simulink model "hexa_tilted_SOF_ANSFT"  (R2023a)
settings: Solver=ode4  StartTime=0.0  StopTime=72  FixedStep=0.01  RelTol=1e-3
model workspace (MAT data in the model file):
  hover_2m = [0  0  0  0  0  0; 0  0  0  0  0  0; 2  2  2  2  2  2; 0  0  0  0  0  0; 0  0  0  0  0  0; 0  0  0  0  0  0]
  square = [0  0  0  0  0  0; 0  0  0  0  0  0; 2.5  2.5  2.5  2.5  2.5  0; 0  0  0  0  0  0; 0  0  0  0  0  0; 0  0  0  0  0  0]
  tf = Simulink.Parameter
  tf.Value = 60
  tf.DataType = 'auto'
  tf.Complexity = 'real'
  tf.Dimensions = [1 1]
  tray0 = [0  0  0  0  0  0; 0  0  0  0  0  0; 0  5  5  5  5  0; 0  0  0  0  0  0; 0  0  0  0  0  0; 0  0  0  0  0  0]
  tray1 = [0  0  0  0  0  0; 0  0  0  0  0  0; 0  2  1  -1  1  2; 0  0  0  0  0  0; 0  0  0  0  0  0; 0  0  0  0  0  0]
  tray2 = [0  2  2  -2  -2  0; 0  0  -2  -2  2  0; 0  2  2  2  2  0; 0  0  0  0  0  0; 0  0  0  0  0  0; 0  0  0  0  0  0]
  tray3 = [0  2  2  -2  -2  0; 0  0  -2  -2  2  0; 0  2.5  2.5  2.5  2.5  0; 0  0  0  0  0  0; 0  0  0  0  0  0; 0  0  0.785  1.042  0.785  0]
  tray5 = [0  0  0  0  0  0; 0  0  0  0  0  0; 0  5  2.5  5  2.5  0; 0  0.15  0.15  0  0  0; 0  0  0.15  0.15  0  0; 0  0  0  0  0  0]
  tray_yaw = [0  0  0  0  0  0; 0  0  0  0  0  0; 0  5  2.5  5  2.5  0; 0  0  0  0  0  0; 0  0  0  0  0  0; 0  0  0.785  1.57  1.57  0.785]
  tray_yaw2 = [0  2  2  2  2  0; 0  0  0  0  0  0; 0  0  0  0  0  0; 0  0  0  0  0  0; 0  0  0  0  0  0; 0.785  0.785  1.042  1.042  0.785  0.785]
  tray_yaw3 = [0  2  2  2  2  0; 0  0  0  0  0  0; 0  0  0  0  0  0; 0  0  0  0  0  0; 0  0  0  0  0  0; 1.57079632679  1.57079632679  1.57079632679  1.57079632679  1.57079632679  1.57079632679]
  z_test = [0  0  0  0  0  0; 0  0  0  0  0  0; 0  1  2  1  1.5  2.25; 0  0  0  0  0  0; 0  0  0  0  0  0; 0  0  0  0  0  0]
undefined symbols (not defined in the file or in its folder): F, Light, MIL
libraries: dspsrcs4 x12, simulink x6, robotcorelib x2, aerolibatmos2 x2, sensorgpslib x1, mspsensorlib x1, sharedtransform x1, aerolibwind2 x1, SignalEditorBlockLib x1
settings Model: Creator=adan  LastModifiedBy=adan
settings OptimizationCC: DefaultParameterBehavior=Inlined  EnhancedBackFolding=on  PassReuseOutputArgsAs=Individual arguments  ZeroExternalMemoryAtStartup=off  ZeroInternalMemoryAtStartup=off  OptimizeBlockOrder=speed  DifferentSizesBufferReuse=on  OptimizationCustomize=off  EfficientTunableParamExpr=on
settings DebuggingCC: ParameterTunabilityLossMsg=error
settings SFSimCC: MATLABDynamicMemAlloc=off
settings RTWCC: Description=Embedded Coder  SystemTargetFile=ert.tlc  TemplateMakefile=ert_default_tmf
settings CodeAppCC: ForceParamTrailComments=on  IgnoreCustomStorageClasses=off  OperatorAnnotations=on  SimulinkDataObjDesc=on  SFDataObjDesc=on  InsertBlockDesc=on
settings ERTTargetCC: TargetLangStandard=C99 (ISO)  GenerateSampleERTMain=on  InlinedParameterPlacement=NonHierarchical  ERTCustomFileTemplate=example_file_process.tlc

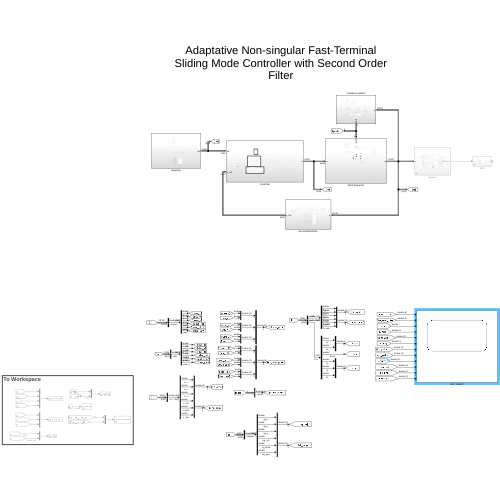
[thumbnail: Simulink's stored preview of the top-level diagram]
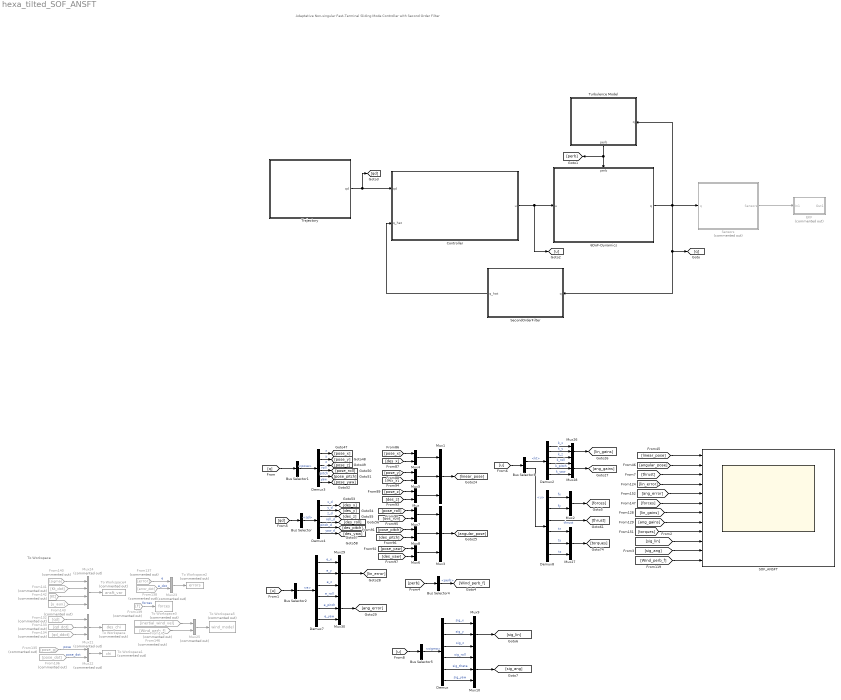
== system hexa_tilted_SOF_ANSFT ==
  note: To Workspace
  note: Adaptative Non-singular Fast-Terminal Sliding Mode Controller with Second Order Filter
  6DoF-Dynamics : Subsystem
      settings: PortSchema="{\"entries\":[{\"content\":{\"sides\":[{\"content\":{\"connectorIds\":[\"In1\"]},\"type\":\"ConnectorPlacement.EquallySpacedRectSide\",\"uuid\":\"d79ec49c-5563-41e0-ac59-6e897bc19fda\"},{\"content\":{\"connectorIds\":[\"Out1\"],\"side\":\"RIGHT\"},\"type\":\"ConnectorPlacement.EquallySpacedRectSide\",\"uuid\":\"1255043e-c90e-4bae-9fb4-4fa06f36f53e\"},{\"content\":{\"connectorIds\":[\"In2\"],\"side\":\"TOP\"},\"type\":\"ConnectorPlacement.EquallySpacedRectSide\",\"uuid\":\"823ada36-3f22-4ee3-87a1-180276f622bc\"}]},\"type\":\"ConnectorPlacement.EquallySpacedConnector\",\"uuid\":\"7403b609-b333-4977-a854-ed7a71f74338\"}],\"packageUris\":[\"http://schema.mathworks.com/mf0/Connector/R2020b\"],\"version\":\"1.0\"}"
  Bus Selector : BusSelector  OutputSignals=qd
  Bus Selector1 : BusSelector  OutputSignals=pose
  Bus Selector2 : BusSelector  OutputSignals=e
  Bus Selector3 : BusSelector  OutputSignals=kt,u
  Bus Selector4 : BusSelector  OutputSignals=perb
  Bus Selector5 : BusSelector  OutputSignals=sigma
  Controller : Subsystem
  Demux{,2..4,7..8} (6 alike) : Demux  Outputs=6
  EKF : Subsystem  Commented=on
  From132 : From  Commented=on  GotoTag=qd
  From133 : From  Commented=on  GotoTag=qd_dot
  From134 : From  Commented=on  GotoTag=qd_ddot
  From135 : From  Commented=on  GotoTag=pose_g
  From136 : From  Commented=on  GotoTag=pose_dot
  From137 : From  Commented=on  GotoTag=error
  From138 : From  Commented=on  GotoTag=error_dot
  From139 : From  Commented=on  GotoTag=F
  From140 : From  Commented=on  GotoTag=sigma
  From141 : From  Commented=on  GotoTag=Kt_dot
  From142 : From  Commented=on  GotoTag=Kt
  From143 : From  Commented=on  GotoTag=u_aux
  From145 : From  Commented=on  GotoTag=inertial_wind_vel
  From146 : From  Commented=on  GotoTag=Wind_perb_f
  Mux{,2,4..8} (7 alike) : Mux  Inputs=2
  Mux{1,3,9..10,26..30} (9 alike) : Mux  Inputs=3
  Mux21 : Mux  Commented=on  Inputs=3
  Mux22 : Mux  Commented=on  Inputs=2
  Mux23 : Mux  Commented=on  Inputs=2
  Mux24 : Mux  Commented=on
  Mux25 : Mux  Commented=on  Inputs=2
  SOF_ANSFT : Scope  NumInputPorts=12
  SecondOrderFilter : Subsystem
      settings: PortSchema="{\"entries\":[{\"content\":{\"sides\":[{\"content\":{\"connectorIds\":[\"Out1\"]},\"type\":\"ConnectorPlacement.EquallySpacedRectSide\",\"uuid\":\"b4c8c2cb-3651-490a-ad01-89b97c3933b2\"},{\"content\":{\"connectorIds\":[\"In1\"],\"side\":\"RIGHT\"},\"type\":\"ConnectorPlacement.EquallySpacedRectSide\",\"uuid\":\"f3956ee2-2beb-41a9-b697-53efa6c7f661\"},{\"content\":{\"side\":\"TOP\"},\"type\":\"ConnectorPlacement.EquallySpacedRectSide\",\"uuid\":\"338fc46d-6a44-4c7a-9eb5-4ab91a191b04\"}]},\"type\":\"ConnectorPlacement.EquallySpacedConnector\",\"uuid\":\"d4e003fa-30a1-40f4-b71f-e0999cd1b71b\"}],\"packageUris\":[\"http://schema.mathworks.com/mf0/Connector/R2020b\"],\"version\":\"1.0\"}"
  Sensors : Subsystem  Commented=on
  To Workspace : ToWorkspace  Commented=on  VariableName=des_chi  SaveFormat=Structure With Time  SampleTime=-1
  To Workspace1 : ToWorkspace  Commented=on  VariableName=chi  SaveFormat=Structure With Time  SampleTime=-1
  To Workspace2 : ToWorkspace  Commented=on  VariableName=errors  SaveFormat=Structure With Time  SampleTime=-1
  To Workspace3 : ToWorkspace  Commented=on  VariableName=forces  SaveFormat=Structure With Time  SampleTime=-1
  To Workspace4 : ToWorkspace  Commented=on  VariableName=ansft_var  SaveFormat=Structure With Time  SampleTime=-1
  To Workspace5 : ToWorkspace  Commented=on  VariableName=wind_model  SaveFormat=Structure With Time  SampleTime=-1
  Trajectory : Subsystem
  Turbulence Model : Subsystem
      settings: PortSchema="{\"entries\":[{\"content\":{\"sides\":[{\"content\":{},\"type\":\"ConnectorPlacement.EquallySpacedRectSide\",\"uuid\":\"1a11629b-61d3-4a8e-8df8-8509e014e579\"},{\"content\":{\"connectorIds\":[\"In1\"],\"side\":\"RIGHT\"},\"type\":\"ConnectorPlacement.EquallySpacedRectSide\",\"uuid\":\"4b15c564-9714-4da5-9436-a08c0d95800f\"},{\"content\":{\"side\":\"TOP\"},\"type\":\"ConnectorPlacement.EquallySpacedRectSide\",\"uuid\":\"dd21b825-2def-4360-b27b-b8c6f475bfab\"},{\"content\":{\"connectorIds\":[\"Out1\"],\"side\":\"BOTTOM\"},\"type\":\"ConnectorPlacement.EquallySpacedRectSide\",\"uuid\":\"594b79ea-4a45-43b1-b592-64a34d0135fb\"}]},\"type\":\"ConnectorPlacement.EquallySpacedConnector\",\"uuid\":\"4c6e67eb-825c-4dd0-a48b-2afa68ae74f5\"}],\"packageUris\":[\"http://schema.mathworks.com/mf0/Connector/R2020b\"],\"version\":\"1.0\"}"
  wires:
  Bus Selector/1 -> Demux4/1  "<qd>"
  Bus Selector1/1 -> Demux3/1  "<pose>"
  Demux3/1 -> [pose_x]  "x"
  Demux3/2 -> [pose_y]  "y"
  Demux3/3 -> [pose_z]  "z"
  Demux3/4 -> [pose_roll]  "roll"
  Demux3/6 -> [pose_yaw]  "yaw"
  Demux3/5 -> [pose_pitch]  "pitch"
  Demux4/6 -> [des_yaw]  "yaw_d"
  Demux4/5 -> [des_pitch]  "pitch_d"
  Demux4/3 -> [des_z]  "z_d"
  Demux4/1 -> [des_x]  "x_d"
  Demux4/4 -> [des_roll]  "roll_d"
  Demux4/2 -> [des_y]  "y_d"
  [pose_x] -> Mux4/1
  [des_x] -> Mux4/2
  [pose_y] -> Mux5/1
  [pose_z] -> Mux/1
  [pose_roll] -> Mux7/1
  [pose_pitch] -> Mux8/1
  [pose_yaw] -> Mux6/1
  [des_y] -> Mux5/2
  [des_z] -> Mux/2
  [des_roll] -> Mux7/2
  [des_pitch] -> Mux8/2
  [des_yaw] -> Mux6/2
  [Wind_perb_f] -> SOF_ANSFT/12
  From133/1 -> Mux21/2
  From132/1 -> Mux21/1
  From134/1 -> Mux21/3
  Mux21/1 -> To Workspace/1
  From136/1 -> Mux22/2  "pose_dot"
  From135/1 -> Mux22/1  "pose"
  Mux22/1 -> To Workspace1/1
  From137/1 -> Mux23/1  "e"
  From138/1 -> Mux23/2  "e_dot"
  Mux23/1 -> To Workspace2/1
  From139/1 -> To Workspace3/1  "forces"
  From140/1 -> Mux24/1
  From141/1 -> Mux24/2
  From142/1 -> Mux24/3
  From143/1 -> Mux24/4
  Mux24/1 -> To Workspace4/1
  From145/1 -> Mux25/1
  From146/1 -> Mux25/2
  Mux25/1 -> To Workspace5/1
  Mux4/1 -> Mux1/1
  Mux/1 -> Mux1/3
  Mux5/1 -> Mux1/2
  Mux1/1 -> [linear_pose]
  Mux7/1 -> Mux3/1
  Mux6/1 -> Mux3/3
  Mux8/1 -> Mux3/2
  [linear_pose] -> SOF_ANSFT/1
  [angular_pose] -> SOF_ANSFT/2
  Demux2/5 -> Mux28/2  "k_pitch"
  Demux2/1 -> Mux26/1  "k_x"
  Demux2/6 -> Mux28/3  "k_yaw"
  Demux2/4 -> Mux28/1  "k_roll"
  Demux2/2 -> Mux26/2  "k_y"
  Demux2/3 -> Mux26/3  "k_z"
  Mux26/1 -> [lin_gains]
  Mux28/1 -> [ang_gains]
  [lin_gains] -> SOF_ANSFT/7
  [ang_gains] -> SOF_ANSFT/8
  Bus Selector3/2 -> Demux8/1  "<u>"
  Demux8/4 -> Mux27/1  "tx"
  Demux8/6 -> Mux27/3  "tz"
  Demux8/3 -> [thrust]  "thrust"
  Demux8/1 -> Mux2/1  "fx"
  Demux8/5 -> Mux27/2  "ty"
  Mux27/1 -> [torques]
  Demux8/2 -> Mux2/2  "fy"
  [forces] -> SOF_ANSFT/6
  [torques] -> SOF_ANSFT/9
  Demux7/5 -> Mux30/2  "e_pitch"
  Bus Selector2/1 -> Demux7/1  "<e>"
  Demux7/2 -> Mux29/2  "e_y"
  Demux7/1 -> Mux29/1  "e_x"
  Mux29/1 -> [lin_error]
  Demux7/3 -> Mux29/3  "e_z"
  Demux7/6 -> Mux30/3  "e_yaw"
  Mux30/1 -> [ang_error]
  Demux7/4 -> Mux30/1  "e_roll"
  [lin_error] -> SOF_ANSFT/4
  [ang_error] -> SOF_ANSFT/5
  Trajectory/1(qd) -> [qd], Controller/1(qd)
  Controller/1(u) -> [u], 6DoF-Dynamics/1(u)
  6DoF-Dynamics/1(q) -> Sensors/1(q), Turbulence Model/1(q), SecondOrderFilter/1(q), [q]
  Turbulence Model/1(perb) -> [perb], 6DoF-Dynamics/2(perb)
  [qd] -> Bus Selector/1
  [q] -> Bus Selector1/1
  [u] -> Bus Selector2/1
  [u] -> Bus Selector3/1
  Bus Selector3/1 -> Demux2/1  "<kt>"
  [perb] -> Bus Selector4/1
  Bus Selector4/1 -> [Wind_perb_f]  "<perb>"
  Mux2/1 -> [forces]
  [thrust] -> SOF_ANSFT/3
  [u] -> Bus Selector5/1
  Mux3/1 -> [angular_pose]
  Bus Selector5/1 -> Demux/1  "<sigma>"
  Demux/1 -> Mux9/1  "sig_x"
  Demux/2 -> Mux9/2  "sig_y"
  Demux/3 -> Mux9/3  "sig_z"
  Demux/5 -> Mux10/2  "sig_theta"
  Demux/4 -> Mux10/1  "sig_roll"
  Demux/6 -> Mux10/3  "sig_yaw"
  Mux9/1 -> [sig_lin]
  Mux10/1 -> [sig_ang]
  [sig_lin] -> SOF_ANSFT/10
  [sig_ang] -> SOF_ANSFT/11
  Sensors/1(Sensors) -> EKF/1(In1)
  SecondOrderFilter/1(q_hat) -> Controller/2(q_hat)

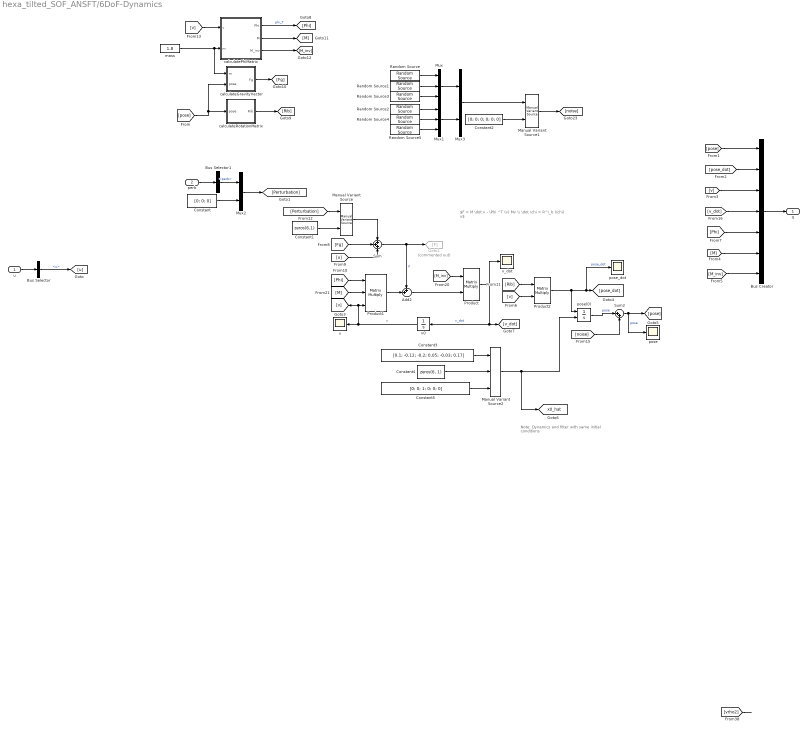
== system hexa_tilted_SOF_ANSFT/6DoF-Dynamics ==
  note: Note: Dynamics and filter with
      | same initial conditions
  note: $F = M \dot v - \Phi ^T (v) Mv \\ \dot \chi = R^i_b (\chi) v$
  u : Inport
  perb : Inport  Port=2
  Add2 : Sum  Inputs=++|
  Bus Creator : BusCreator  Inputs=7
  Bus Selector : BusSelector  OutputSignals=u
  Bus Selector1 : BusSelector  OutputSignals=perb
  Constant : Constant  Value=[0; 0; 0]
  Constant1 : Constant  Value=zeros(6,1)
  Constant2 : Constant  Value=[0; 0; 0; 0; 0; 0]
  Constant3 : Constant  Value=[0.1; -0.12; -0.2; 0.05; -0.03; 0.17]
  Constant4 : Constant  Value=zeros(6, 1)
  Constant5 : Constant  Value=[0; 0; 1; 0; 0; 0]
  Goto2 : Goto  Commented=on  GotoTag=F
  Manual Variant Source : simulink/Signal Routing/Manual Variant Source  NumChoices=2  LabelModeActiveChoice=V_1
  Manual Variant Source1 : simulink/Signal Routing/Manual Variant Source  NumChoices=2  LabelModeActiveChoice=V_1
  Manual Variant Source2 : simulink/Signal Routing/Manual Variant Source  NumChoices=3  LabelModeActiveChoice=V_2
  Mux : Mux  Inputs=3
  Mux1 : Mux  Inputs=3
  Mux2 : Mux  Inputs=2
  Mux3 : Mux  Inputs=2
  Product : Product  Multiplication=Matrix(*)
  Product1 : Product  Inputs=3  Multiplication=Matrix(*)
  Product2 : Product  Multiplication=Matrix(*)
  Random Source : dspsrcs4/Random Source  SrcType=Gaussian  NormMethod=Ziggurat  CltLength=12  MinVal=0  MaxVal=1  MeanVal=0.005  VarVal=0.001 * 0.001  RepMode=Not repeatable  rawSeed=1  IsInherit=off  SampMode=Continuous  SampTime=0.01  SampFrame=1  DataType=Double  OutComplex=Real  OutputFrames=off
  Random Source1 : dspsrcs4/Random Source  SrcType=Gaussian  NormMethod=Ziggurat  CltLength=12  MinVal=0  MaxVal=1  MeanVal=0.005  VarVal=0.001 * 0.001  RepMode=Not repeatable  rawSeed=1  IsInherit=off  SampMode=Continuous  SampTime=0.01  SampFrame=1  DataType=Double  OutComplex=Real  OutputFrames=off
  Random Source2 : dspsrcs4/Random Source  SrcType=Gaussian  NormMethod=Ziggurat  CltLength=12  MinVal=0  MaxVal=1  MeanVal=0.001  VarVal=0.001 * 0.001  RepMode=Not repeatable  rawSeed=1  IsInherit=off  SampMode=Continuous  SampTime=0.01  SampFrame=1  DataType=Double  OutComplex=Real  OutputFrames=off
  Random Source3 : dspsrcs4/Random Source  SrcType=Gaussian  NormMethod=Ziggurat  CltLength=12  MinVal=0  MaxVal=1  MeanVal=0.005  VarVal=0.001 * 0.001  RepMode=Not repeatable  rawSeed=1  IsInherit=off  SampMode=Continuous  SampTime=0.01  SampFrame=1  DataType=Double  OutComplex=Real  OutputFrames=off
  Random Source4 : dspsrcs4/Random Source  SrcType=Gaussian  NormMethod=Ziggurat  CltLength=12  MinVal=0  MaxVal=1  MeanVal=0.001  VarVal=0.001 * 0.001  RepMode=Not repeatable  rawSeed=1  IsInherit=off  SampMode=Continuous  SampTime=0.01  SampFrame=1  DataType=Double  OutComplex=Real  OutputFrames=off
  Random Source5 : dspsrcs4/Random Source  SrcType=Gaussian  NormMethod=Ziggurat  CltLength=12  MinVal=0  MaxVal=1  MeanVal=0.001  VarVal=0.001 * 0.001  RepMode=Not repeatable  rawSeed=1  IsInherit=off  SampMode=Continuous  SampTime=0.01  SampFrame=1  DataType=Double  OutComplex=Real  OutputFrames=off
  Sum : Sum  Inputs=+++
  Sum2 : Sum  Inputs=|++
  calculateGravityVector : MATLAB Function  TreatAsAtomicUnit=on
  calculatePhiMatrix : MATLAB Function  TreatAsAtomicUnit=on
  calculateRotationMatrix : MATLAB Function  TreatAsAtomicUnit=on
  mass : Constant  Value=1.8
  pose : Scope
  pose(0) : Integrator  InitialConditionSource=external  InitialCondition=[0; 0; 0; 0.05; -0.03; 0.12]
  pose_dot : Scope
  v : Scope
  v0 : Integrator  InitialCondition=[0; 0; 0; 0; 0; 0]
  v_dot : Scope
  q : Outport
  tag scope: x0_hat=global
  wires:
  [M_inv] -> Product/1
  Product1/1 -> Add2/2
  [v] -> Product2/2
  Add2/1 -> Product/2
  Product/1 -> v_dot/1, [v_dot], v0/1  "v_dot"
  Product2/1 -> pose(0)/1, pose_dot/1, [pose_dot]  "pose_dot"
  [M] -> Product1/2
  [Rib] -> Product2/1
  [Phi] -> Product1/1
  [v] -> calculatePhiMatrix/1(v)
  calculatePhiMatrix/2(M) -> [M]
  calculatePhiMatrix/1(Phi) -> [Phi]  "phi_T"
  calculatePhiMatrix/3(M_inv) -> [M_inv]
  calculateRotationMatrix/1(Rib) -> [Rib]
  [pose] -> calculateRotationMatrix/1(pose), calculateGravityVector/2(pose)
  u/1 -> Bus Selector/1
  [pose] -> Bus Creator/1
  [pose_dot] -> Bus Creator/2
  [v] -> Bus Creator/3
  Bus Creator/1 -> q/1
  [Phi] -> Bus Creator/5
  [M] -> Bus Creator/6
  [M_inv] -> Bus Creator/7
  [Fg] -> Sum/2
  perb/1 -> Bus Selector1/1
  Bus Selector/1 -> [u]  "<u>"
  Bus Selector1/1 -> Mux2/1  "<perb>"
  Constant/1 -> Mux2/2
  Mux2/1 -> [Perturbation]
  [Perturbation] -> Manual Variant Source/1
  Sum/1 -> Goto2/1, Add2/1  "F"
  v0/1 -> [v], Product1/3, v/1  "v"
  pose(0)/1 -> Sum2/1  "pose"
  Sum2/1 -> pose/1, [pose]  "pose"
  [noise] -> Sum2/2
  [v_dot] -> Bus Creator/4
  [u] -> Sum/3
  Manual Variant Source/1 -> Sum/1
  Constant1/1 -> Manual Variant Source/2
  [vrho2] -> ?
  ? -> ?
  calculateGravityVector/1(Fg) -> [Fg]
  mass/1 -> calculateGravityVector/1(m), calculatePhiMatrix/2(m)
  Manual Variant Source1/1 -> [noise]
  Constant2/1 -> Manual Variant Source1/2
  Random Source/1 -> Mux/1
  Random Source1/1 -> Mux/2
  Random Source2/1 -> Mux1/1
  Random Source3/1 -> Mux/3
  Random Source4/1 -> Mux1/2
  Random Source5/1 -> Mux1/3
  Mux/1 -> Mux3/1
  Mux1/1 -> Mux3/2
  Mux3/1 -> Manual Variant Source1/1
  Constant3/1 -> Manual Variant Source2/1
  Constant4/1 -> Manual Variant Source2/2
  Manual Variant Source2/1 -> [x0_hat], pose(0)/2
  Constant5/1 -> Manual Variant Source2/3

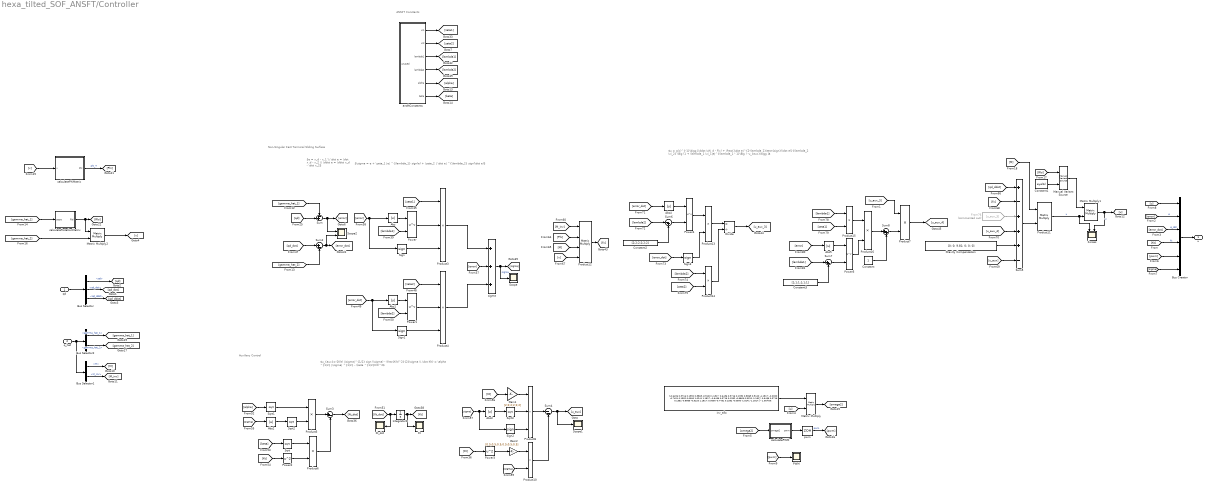
== system hexa_tilted_SOF_ANSFT/Controller ==
  note: $u = g(x)^{-1}\bigg [\ddot \chi_d - f(x) + \frac{|\dot e|^{2-\lambda_2}\text{sign}(\dot e)}{\lambda_2 \xi_2} \Big (1 + \lambda_1 \xi_1|e|^{\lambda_1 - 1}\Big ) -u_{aux}\bigg ]$
  note: Auxiliary Control
  note: Non-Singular Fast Terminal Sliding Surface
  note: $e = x_d - x_1 \\ \dot e = \dot x_d - x_2 \\ \ddot e = \ddot x_d - \dot x_2$
  note: $\sigma = e + \zeta_1 |e| ^{\lambda_1} sign(e) + \zeta_2 | \dot e| ^{\lambda_2} sign(\dot e)$
  note: $u_{aux}=-2K(t) |\sigma|^{1/2} sign (\sigma) - \frac{K(t)^2}{2}\sigma \\ \dot K(t) = \alpha ^{1/2} |\sigma| ^{1/2} - \beta ^{1/2}K(t)^2$
  note: ANSFT Constants
  qd : Inport
  q_hat : Inport  Port=2
  Abs{,1..5} (6 alike) : Abs  SaturateOnIntegerOverflow=off
  Bus Creator : BusCreator  Inputs=6
  Bus Selector : BusSelector  OutputSignals=qd,qd_dot,qd_ddot
  Bus Selector1 : BusSelector  OutputSignals=M,M_inv
  Bus Selector2 : BusSelector  OutputSignals=gamma_hat_1,gamma_hat_2
  Constant : Constant
  Constant1 : Constant  Value=eye(6)
  Constant2 : Constant  Value=[2;2;2;2;2;2]
  Constant3 : Constant  Value=[1;1;1;1;1;1]
  Divide : Product  Inputs=*/
  Forces : Scope  NumInputPorts=2
  From76 : From  Commented=on  GotoTag=u_aux_3
  Gain1 : Gain  Gain=[2;2;2;2;2;2]
  Gain2 : Gain  Gain=[0.5;0.5;0.5;0.5;0.5;0.5]
  Gravity Compensation : Constant  Value=[0; 0; 9.81; 0; 0; 0]
  Integrator2 : Integrator  InitialCondition=[0;0;0;0;0;0]
  Kt : Scope
  Kt_dot : Scope
  Manual Variant Source : simulink/Signal Routing/Manual Variant Source  NumChoices=2  LabelModeActiveChoice=V_2
  Matrix Multiply : Product  Multiplication=Matrix(*)
  Matrix Multiply1 : Product  Multiplication=Matrix(*)
  Matrix Multiply2 : Product  Multiplication=Matrix(*)
  PWM : Scope
  Power{,1,4..5} (4 alike) : Math  Operator=pow
  Power2 : Math  Operator=square
  Power3 : Math  Operator=square
  Product{5..7,10,13..16} (8 alike) : Product
  Product11 : Product  Multiplication=Matrix(*)
  Product12 : Product  Inputs=4  Multiplication=Matrix(*)
  Product3 : Product  Inputs=3
  Product4 : Product  Inputs=3
  Product8 : Product  Inputs=3
  Scope : Scope
  Scope1 : Scope
  Scope2 : Scope  NumInputPorts=2
  Sign{,1..3} (4 alike) : Signum
  Sqrt{,1..3} (4 alike) : Sqrt
  Sum : Sum  Inputs=-+|
  Sum2 : Sum  Inputs=|+-
  Sum3 : Sum  Inputs=|+-
  Sum4 : Sum  Inputs=|--
  Sum5 : Sum  Inputs=+-+++-
  Sum6 : Sum  Inputs=|-+
  Sum7 : Sum  Inputs=|+-
  Sum8 : Sum  Inputs=|++
  ansftConstants : MATLAB Function  TreatAsAtomicUnit=on
  calculatePWM : MATLAB Function  TreatAsAtomicUnit=on
  calculatePhiMatrix : MATLAB Function  TreatAsAtomicUnit=on
  calculateRotationMatrix : MATLAB Function  TreatAsAtomicUnit=on
  inv_allo : Constant  Value=|
      | [-0.6436    0.3716    0.1352    0.8869   -0.5120    1.1817;
      |             0.6436    0.3716    0.1352    0.8869    0.5120   -1.1817;
      |             -0.0000   -0.7431    0.1352    0.0000    1.0241    1.1817;
      |             -0.6436    0.3716    0.1352   -0.8869    0.5120   -1.1817;
      |             0.6436    0.3716    0.1352   -0.8869   -0.5120    1.1817;
      |             0.0000   -0.7431    0.1352   -0.0000   -1.0241   -1.1817;] * 1.0e+05;
  pwm : ZeroOrderHold  SampleTime=-1
  sigma : Sum  Inputs=+++
  u : Outport
  wires:
  Product6/1 -> Sum3/2
  [M_inv] -> Product12/1
  Sign1/1 -> Product4/3
  Sum8/1 -> Product7/2
  Product5/1 -> Sum3/1
  [error_dot] -> Abs4/1
  [fx] -> Sum5/2
  [u_aux_3] -> Product7/1
  Power5/1 -> Product16/2
  [zeta1] -> Product3/1
  Constant/1 -> Sum8/2
  Product16/1 -> Sum8/1
  Sqrt/1 -> Product6/1
  Product10/1 -> Sum4/2
  Sum6/1 -> Power4/2
  Product15/1 -> Product16/1
  [qd_ddot] -> Sum5/1
  [lambda2] -> Sum6/1
  Sum4/1 -> Scope1/1, [u_aux]
  [Kt] -> Power2/1
  Gain1/1 -> Product8/1
  Sum5/1 -> Product11/2
  From76/1 -> Sum5/3
  Sqrt1/1 -> Product5/1
  Constant2/1 -> Sum6/2
  Sign3/1 -> Product13/2
  [lambda1] -> Sum7/1
  Power3/1 -> Gain2/1
  Product3/1 -> sigma/1
  [beta] -> Sqrt/1
  Abs4/1 -> Power4/1
  [Kt] -> Gain1/1
  [error_dot] -> Sign1/1, Abs1/1
  Divide/1 -> [u_aux_3]
  [u_aux_4] -> Sum5/4
  [sigma] -> Sign2/1, Abs3/1
  [zeta2] -> Product14/2
  Sum3/1 -> [Kt_dot]
  Product12/1 -> [fx]
  Product8/1 -> Sum4/1
  [sigma] -> Abs2/1
  Power/1 -> Product3/2
  Product4/1 -> sigma/3
  [u_aux] -> Sum5/6
  Constant3/1 -> Sum7/2
  [error] -> sigma/2
  Abs3/1 -> Sqrt3/1
  [alpha] -> Sqrt1/1
  Sum7/1 -> Power5/2
  Sqrt2/1 -> Product5/2
  Power4/1 -> Product13/1
  [M] -> Product11/1
  sigma/1 -> Scope/1, [sigma]  "sigma"
  Sign/1 -> Product3/3
  Abs2/1 -> Sqrt2/1
  [M] -> Product12/3
  [Kt_dot] -> Kt_dot/1, Integrator2/1
  Power1/1 -> Product4/2
  [lambda2] -> Product14/1
  Power2/1 -> Product6/2
  [zeta1] -> Product15/2
  [Kt] -> Power3/1
  [lambda1] -> Product15/1
  [error_dot] -> Sign3/1
  Sqrt3/1 -> Product8/2
  Product13/1 -> Divide/1
  [zeta2] -> Product4/1
  Integrator2/1 -> Kt/1, [Kt]
  [Phi] -> Product12/2
  Abs/1 -> Power/1
  Abs1/1 -> Power1/1
  [v] -> Product12/4
  Sum2/1 -> Scope2/2, [error_dot]
  Sum/1 -> Scope2/1, [error]
  Gain2/1 -> Product10/1
  Product14/1 -> Divide/2
  Gravity Compensation/1 -> Sum5/5
  [lambda2] -> Power1/2
  [error] -> Abs5/1
  Abs5/1 -> Power5/1
  Product7/1 -> [u_aux_4]
  [sigma] -> Product10/2
  [lambda1] -> Power/2
  Sign2/1 -> Product8/3
  [error] -> Sign/1, Abs/1
  [qd_dot] -> Sum2/1
  Bus Creator/1 -> u/1
  ansftConstants/3(lambda1) -> [lambda1]
  ansftConstants/1(xi1) -> [zeta1]
  ansftConstants/2(xi2) -> [zeta2]
  ansftConstants/5(alpha) -> [alpha]
  ansftConstants/6(beta) -> [beta]
  ansftConstants/4(lambda2) -> [lambda2]
  qd/1 -> Bus Selector/1
  Bus Selector/2 -> [qd_dot]  "<qd_dot>"
  Bus Selector/1 -> [qd]  "<qd>"
  Bus Selector/3 -> [qd_ddot]  "<qd_ddot>"
  q_hat/1 -> Bus Selector1/1, Bus Selector2/1
  Product11/1 -> Forces/1, Matrix Multiply1/2  "u"
  [error] -> Bus Creator/2  "e"
  [error_dot] -> Bus Creator/3  "e_dot"
  [Kt] -> Bus Creator/4  "kt"
  inv_allo/1 -> Matrix Multiply/1
  [u] -> Matrix Multiply/2
  Matrix Multiply/1 -> [omega2]
  [omega2] -> calculatePWM/1(omega2)
  calculatePWM/1(pwm) -> pwm/1
  pwm/1 -> [pwm]  "pwm"
  [pwm] -> Bus Creator/5
  [sigma] -> Bus Creator/6
  [u] -> Bus Creator/1
  [pwm] -> PWM/1
  Matrix Multiply1/1 -> Forces/2, [u]  "u"
  [Rbi] -> Manual Variant Source/1
  Constant1/1 -> Manual Variant Source/2
  Manual Variant Source/1 -> Matrix Multiply1/1
  Bus Selector2/2 -> [gamma_hat_2]  "<gamma_hat_2>"
  Bus Selector2/1 -> [gamma_hat_1]  "<gamma_hat_1>"
  [gamma_hat_2] -> Sum2/2
  [qd] -> Sum/2
  [gamma_hat_1] -> Sum/1
  Bus Selector1/2 -> [M_inv]  "<M_inv>"
  Bus Selector1/1 -> [M]  "<M>"
  calculatePhiMatrix/1(Phi) -> [Phi]  "phi_T"
  [v] -> calculatePhiMatrix/1(v)
  calculateRotationMatrix/1(Rbi) -> Matrix Multiply2/1, [Rbi]
  [gamma_hat_1] -> calculateRotationMatrix/1(pose)
  [gamma_hat_2] -> Matrix Multiply2/2
  Matrix Multiply2/1 -> [v]

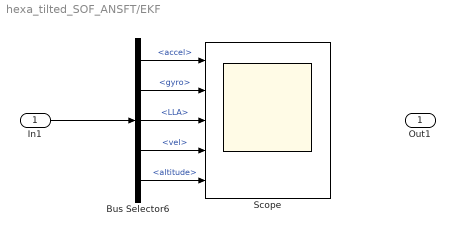
== system hexa_tilted_SOF_ANSFT/EKF ==
  In1 : Inport
  Bus Selector6 : BusSelector  OutputSignals=signal1.accel,signal1.gyro,signal2.LLA,signal2.vel,altitude
  Scope : Scope  NumInputPorts=5
  Out1 : Outport
  wires:
  In1/1 -> Bus Selector6/1
  Bus Selector6/1 -> Scope/1  "<accel>"
  Bus Selector6/2 -> Scope/2  "<gyro>"
  Bus Selector6/4 -> Scope/4  "<vel>"
  Bus Selector6/3 -> Scope/3  "<LLA>"
  Bus Selector6/5 -> Scope/5  "<altitude>"

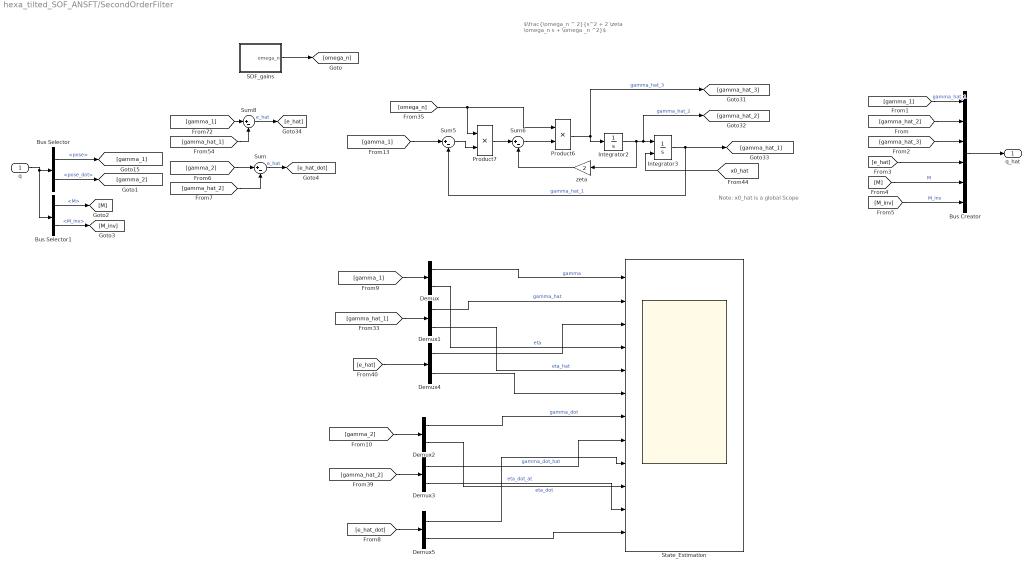
== system hexa_tilted_SOF_ANSFT/SecondOrderFilter ==
  note: Note: x0_hat is a global Scope
  note: $\frac{\omega_n ^ 2}{s^2 + 2 \zeta \omega_n s + \omega _n ^2}$
  q : Inport
  Bus Creator : BusCreator  Inputs=6
  Bus Selector : BusSelector  OutputSignals=pose,pose_dot
  Bus Selector1 : BusSelector  OutputSignals=M,M_inv
  Demux{,1..5} (6 alike) : Demux  Outputs=2
  Integrator2 : Integrator
  Integrator3 : Integrator  InitialConditionSource=external
  Product6 : Product
  Product7 : Product
  SOF_gains : MATLAB Function  TreatAsAtomicUnit=on
  State_Estimation : Scope  NumInputPorts=12
  Sum{,5..6,8} (4 alike) : Sum  Inputs=|+-
  zeta : Gain  Gain=2
  q_hat : Outport
  wires:
  [gamma_1] -> Sum5/1
  Integrator3/1 -> [gamma_hat_1], Sum5/2  "gamma_hat_1"
  zeta/1 -> Sum6/2
  Sum8/1 -> [e_hat]  "e_hat"
  [omega_n] -> Product7/1, Product6/1
  Sum6/1 -> Product6/2
  Product6/1 -> Integrator2/1, [gamma_hat_3]  "gamma_hat_3"
  Integrator2/1 -> zeta/1, [gamma_hat_2], Integrator3/1  "gamma_hat_2"
  [gamma_1] -> Sum8/1
  [x0_hat] -> Integrator3/2
  Sum5/1 -> Product7/2
  Product7/1 -> Sum6/1
  [gamma_hat_1] -> Sum8/2
  q/1 -> Bus Selector1/1, Bus Selector/1
  Bus Selector/1 -> [gamma_1]  "<pose>"
  SOF_gains/1(omega_n) -> [omega_n]
  [gamma_1] -> Bus Creator/1  "gamma_hat_1"
  [gamma_hat_2] -> Bus Creator/2
  [gamma_hat_3] -> Bus Creator/3
  [e_hat] -> Bus Creator/4
  Bus Creator/1 -> q_hat/1
  Bus Selector1/1 -> [M]  "<M>"
  Bus Selector1/2 -> [M_inv]  "<M_inv>"
  [M] -> Bus Creator/5  "M"
  [M_inv] -> Bus Creator/6  "M_inv"
  Bus Selector/2 -> [gamma_2]  "<pose_dot>"
  [gamma_2] -> Sum/1
  [gamma_hat_2] -> Sum/2
  Sum/1 -> [e_hat_dot]  "e_hat"
  Demux5/1 -> State_Estimation/9
  [gamma_hat_2] -> Demux3/1
  Demux1/1 -> State_Estimation/2  "gamma_hat"
  Demux2/2 -> State_Estimation/10  "eta_dot"
  Demux/2 -> State_Estimation/4  "eta"
  [gamma_hat_1] -> Demux1/1
  Demux5/2 -> State_Estimation/12
  Demux3/2 -> State_Estimation/11  "eta_dot_at"
  Demux1/2 -> State_Estimation/5  "eta_hat"
  [gamma_2] -> Demux2/1
  Demux3/1 -> State_Estimation/8  "gamma_dot_hat"
  Demux2/1 -> State_Estimation/7  "gamma_dot"
  [gamma_1] -> Demux/1
  [e_hat] -> Demux4/1
  Demux/1 -> State_Estimation/1  "gamma"
  Demux4/1 -> State_Estimation/3
  [e_hat_dot] -> Demux5/1
  Demux4/2 -> State_Estimation/6

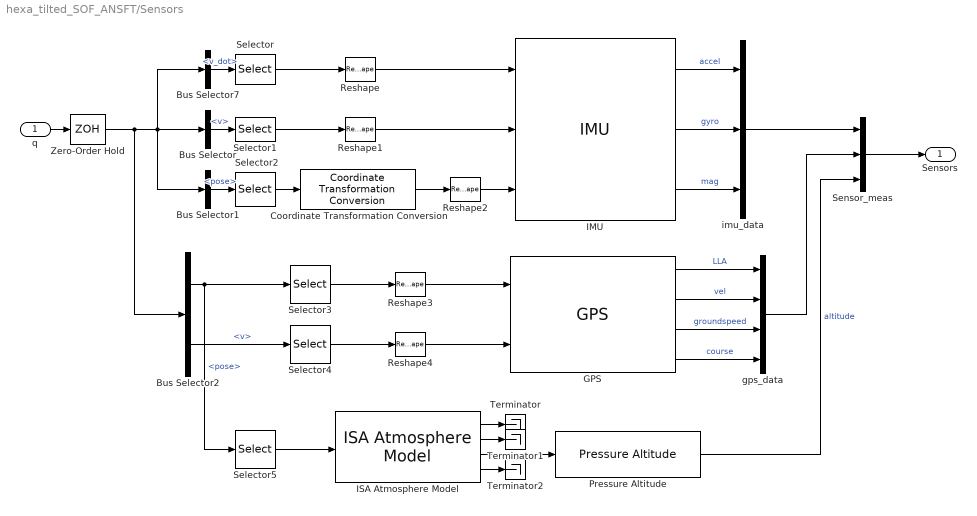
== system hexa_tilted_SOF_ANSFT/Sensors ==
  q : Inport
  Bus Selector : BusSelector  OutputSignals=v
  Bus Selector1 : BusSelector  OutputSignals=pose
  Bus Selector2 : BusSelector  OutputSignals=pose,v
  Bus Selector7 : BusSelector  OutputSignals=v_dot
  Coordinate Transformation Conversion : robotcorelib/Coordinate Transformation Conversion  InputRepresentation=Euler Angles  InputEulerSequence=ZYX  ShowTrVecInputPort=on  OutputRepresentation=Quaternion  OutputEulerSequence=ZYX  ShowTrVecOutputPort=on  SimulateUsing=Interpreted execution
      settings: LibrarySourceBlock=navlib/Utilities/Coordinate Transformation Conversion
  GPS : sensorgpslib/GPS  DispRefFrame=ENU  PositionInputFormat=Local  ReferenceLocation=[ 0, 0, 0 ]  HorizontalPositionAccuracy=1.6  VerticalPositionAccuracy=3  VelocityAccuracy=0.1  DecayFactor=0.999  SeedDouble=67  SimulateUsing=Interpreted execution
      settings: LibrarySourceBlock=mspsensorlib/GPS
  IMU : mspsensorlib/IMU  DispRefFrame=NED  Temperature=25  MagneticFieldNED=[ 27.5550, -2.4169, -16.0849 ]  MagneticFieldENU=[ -2.4169, 27.5550, 16.0849 ]  SeedDouble=67  SimulateUsing=Interpreted execution  AccelParamsMeasurementRange=Inf  AccelParamsResolution=0  AccelParamsConstantBias=[ 0.01, 0.01, 0.01 ]  AccelParamsAxesMisalignment=[ 100, 0, 0; 0, 100, 0; 0, 0, 100 ]  AccelParamsNoiseDensity=[ 0, 0, 0 ]  AccelParamsBiasInstability=[ 0.01, 0.01, 0.01 ]  AccelParamsRandomWalk=[ 0, 0, 0 ]  AccelParamsTemperatureBias=[ 0, 0, 0 ]  AccelParamsTemperatureScaleFactor=[ 0, 0, 0 ]  GyroParamsMeasurementRange=Inf  GyroParamsResolution=0  GyroParamsConstantBias=[ 0.01, 0.01, 0.01 ]  GyroParamsAxesMisalignment=[ 100, 0, 0; 0, 100, 0; 0, 0, 100 ]  GyroParamsAccelerationBias=[ 0, 0, 0 ]  GyroParamsNoiseDensity=[ 0, 0, 0 ]  GyroParamsBiasInstability=[ 0.01, 0.01, 0.01 ]  GyroParamsRandomWalk=[ 0, 0, 0 ]  GyroParamsTemperatureBias=[ 0, 0, 0 ]  GyroParamsTemperatureScaleFactor=[ 0, 0, 0 ]  MagParamsMeasurementRange=Inf  MagParamsResolution=0  MagParamsConstantBias=[ 0, 0, 0 ]  MagParamsAxesMisalignment=[ 100, 0, 0; 0, 100, 0; 0, 0, 100 ]  MagParamsNoiseDensity=[ 0, 0, 0 ]  MagParamsBiasInstability=[ 0, 0, 0 ]  MagParamsRandomWalk=[ 0, 0, 0 ]  MagParamsTemperatureBias=[ 0, 0, 0 ]  MagParamsTemperatureScaleFactor=[ 0, 0, 0 ]
  ISA Atmosphere Model : aerolibatmos2/ISA Atmosphere Model  custom=off  g=9.80665  gamma=1.4  R=287.0531  L=0.0065  h_trop=11000  h_strat=20000  rho0=1.225  P0=101325  T0=288.15  h0=0
  Pressure Altitude : aerolibatmos2/Pressure Altitude  units=Metric (MKS)  action=Warning
  Reshape{,1..4} (5 alike) : Reshape  OutputDimensionality=Row vector (2-D)
  Selector : Selector  InputPortWidth=6  IndexOptions=Index vector (dialog)  Indices=[1:3]  OutputSizes=1
  Selector1 : Selector  InputPortWidth=6  IndexOptions=Index vector (dialog)  Indices=[4:6]  OutputSizes=1
  Selector2 : Selector  InputPortWidth=6  IndexOptions=Index vector (dialog)  Indices=[6 5 4]  OutputSizes=1
  Selector3 : Selector  InputPortWidth=6  IndexOptions=Index vector (dialog)  Indices=[1:3]  OutputSizes=1
  Selector4 : Selector  InputPortWidth=6  IndexOptions=Index vector (dialog)  Indices=[1:3]  OutputSizes=1
  Selector5 : Selector  InputPortWidth=6  IndexOptions=Index vector (dialog)  Indices=[1]  OutputSizes=1
  Sensor_meas : BusCreator  Inputs=3
  Terminator : Terminator
  Terminator1 : Terminator
  Terminator2 : Terminator
  Zero-Order Hold : ZeroOrderHold  SampleTime=0.01
  gps_data : BusCreator  Inputs=4
  imu_data : BusCreator  Inputs=3
  Sensors : Outport
  wires:
  Bus Selector7/1 -> Selector/1  "<v_dot>"
  q/1 -> Zero-Order Hold/1
  Selector/1 -> Reshape/1
  Bus Selector/1 -> Selector1/1  "<v>"
  Selector1/1 -> Reshape1/1
  Bus Selector1/1 -> Selector2/1  "<pose>"
  Selector2/1 -> Coordinate Transformation Conversion/1
  Coordinate Transformation Conversion/1 -> Reshape2/1
  IMU/2 -> imu_data/2  "gyro"
  IMU/1 -> imu_data/1  "accel"
  IMU/3 -> imu_data/3  "mag"
  Reshape1/1 -> IMU/2
  Reshape/1 -> IMU/1
  Reshape2/1 -> IMU/3
  Zero-Order Hold/1 -> Bus Selector2/1, Bus Selector7/1, Bus Selector1/1, Bus Selector/1
  Bus Selector2/1 -> Selector5/1, Selector3/1  "<pose>"
  Bus Selector2/2 -> Selector4/1  "<v>"
  Selector3/1 -> Reshape3/1
  Selector4/1 -> Reshape4/1
  GPS/4 -> gps_data/4  "course"
  GPS/3 -> gps_data/3  "groundspeed"
  GPS/2 -> gps_data/2  "vel"
  GPS/1 -> gps_data/1  "LLA"
  imu_data/1 -> Sensor_meas/1
  gps_data/1 -> Sensor_meas/2
  Sensor_meas/1 -> Sensors/1
  Reshape3/1 -> GPS/1
  Reshape4/1 -> GPS/2
  Selector5/1 -> ISA Atmosphere Model/1
  ISA Atmosphere Model/3 -> Pressure Altitude/1
  ISA Atmosphere Model/1 -> Terminator/1
  ISA Atmosphere Model/2 -> Terminator1/1
  ISA Atmosphere Model/4 -> Terminator2/1
  Pressure Altitude/1 -> Sensor_meas/3  "altitude"

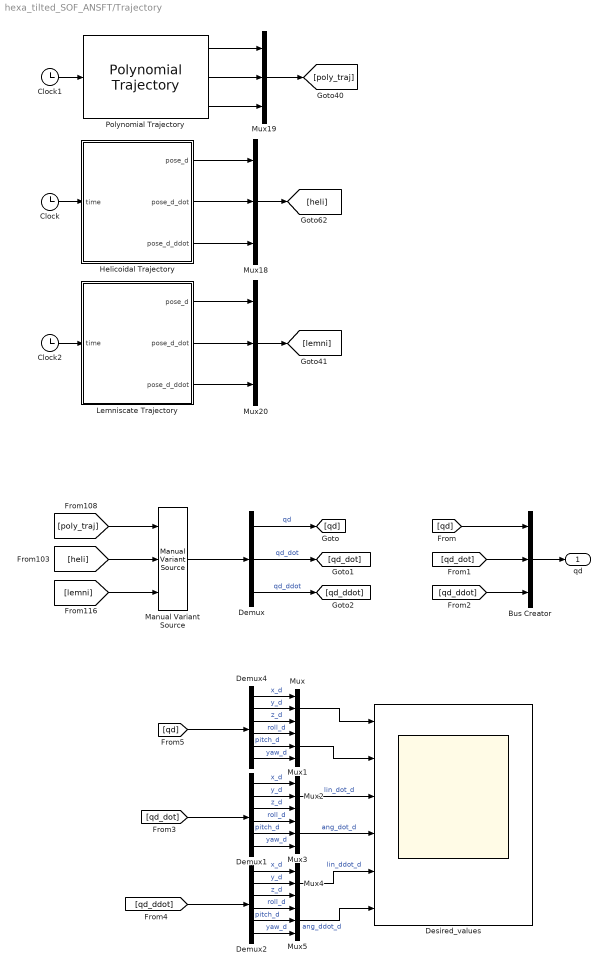
== system hexa_tilted_SOF_ANSFT/Trajectory ==
  Bus Creator : BusCreator  Inputs=3
  Clock : Clock
  Clock1 : Clock
  Clock2 : Clock
  Demux : Demux  Outputs=3
  Demux1 : Demux  Outputs=6
  Demux2 : Demux  Outputs=6
  Demux4 : Demux  Outputs=6
  Desired_values : Scope  NumInputPorts=6
  Helicoidal Trajectory : MATLAB Function  TreatAsAtomicUnit=on
  Lemniscate Trajectory : MATLAB Function  TreatAsAtomicUnit=on
  Manual Variant Source : simulink/Signal Routing/Manual Variant Source  NumChoices=3  LabelModeActiveChoice=V_2
  Mux{,1..5,18..20} (9 alike) : Mux  Inputs=3
  Polynomial Trajectory : robotcorelib/Polynomial Trajectory  WaypointSource=Internal  Waypoints=zeros(6 ,6)  TimePoints=[ 0, 12, 24, 36, 48, tf ]  TimeInterval=[ 1, 4 ]  Method=Cubic Polynomial  ParameterSource=Internal  VelocityBoundaryCondition=zeros( 6, 6 )  AccelerationBoundaryCondition=zeros( 2, 5 )  SimulateUsing=Interpreted execution
  qd : Outport
  wires:
  Lemniscate Trajectory/2(pose_d_dot) -> Mux20/2
  Polynomial Trajectory/3 -> Mux19/3
  Helicoidal Trajectory/1(pose_d) -> Mux18/1
  Clock1/1 -> Polynomial Trajectory/1
  Mux18/1 -> [heli]
  Lemniscate Trajectory/3(pose_d_ddot) -> Mux20/3
  Polynomial Trajectory/2 -> Mux19/2
  Clock2/1 -> Lemniscate Trajectory/1(time)
  Helicoidal Trajectory/3(pose_d_ddot) -> Mux18/3
  Mux19/1 -> [poly_traj]
  Mux20/1 -> [lemni]
  Lemniscate Trajectory/1(pose_d) -> Mux20/1
  Helicoidal Trajectory/2(pose_d_dot) -> Mux18/2
  Clock/1 -> Helicoidal Trajectory/1(time)
  Polynomial Trajectory/1 -> Mux19/1
  Mux3/1 -> Desired_values/4  "ang_dot_d"
  Mux4/1 -> Desired_values/5  "lin_ddot_d"
  Demux1/3 -> Mux2/3  "z_d"
  Demux1/6 -> Mux3/3  "yaw_d"
  Demux2/3 -> Mux4/3  "z_d"
  [qd_dot] -> Bus Creator/2
  Mux5/1 -> Desired_values/6  "ang_ddot_d"
  Demux4/4 -> Mux1/1  "roll_d"
  [lemni] -> Manual Variant Source/3
  Demux2/2 -> Mux4/2  "y_d"
  Demux4/5 -> Mux1/2  "pitch_d"
  Demux4/2 -> Mux/2  "y_d"
  Demux1/4 -> Mux3/1  "roll_d"
  Demux1/2 -> Mux2/2  "y_d"
  Demux/3 -> [qd_ddot]  "qd_ddot"
  Bus Creator/1 -> qd/1
  Demux2/4 -> Mux5/1  "roll_d"
  Demux1/1 -> Mux2/1  "x_d"
  [qd_dot] -> Demux1/1
  [poly_traj] -> Manual Variant Source/1
  Demux2/1 -> Mux4/1  "x_d"
  Mux2/1 -> Desired_values/3  "lin_dot_d"
  Demux2/6 -> Mux5/3  "yaw_d"
  Demux4/6 -> Mux1/3  "yaw_d"
  [heli] -> Manual Variant Source/2
  [qd_ddot] -> Bus Creator/3
  [qd_ddot] -> Demux2/1
  Mux1/1 -> Desired_values/2
  Manual Variant Source/1 -> Demux/1
  Demux4/3 -> Mux/3  "z_d"
  Mux/1 -> Desired_values/1
  [qd] -> Demux4/1
  Demux1/5 -> Mux3/2  "pitch_d"
  Demux4/1 -> Mux/1  "x_d"
  Demux2/5 -> Mux5/2  "pitch_d"
  [qd] -> Bus Creator/1
  Demux/2 -> [qd_dot]  "qd_dot"
  Demux/1 -> [qd]  "qd"

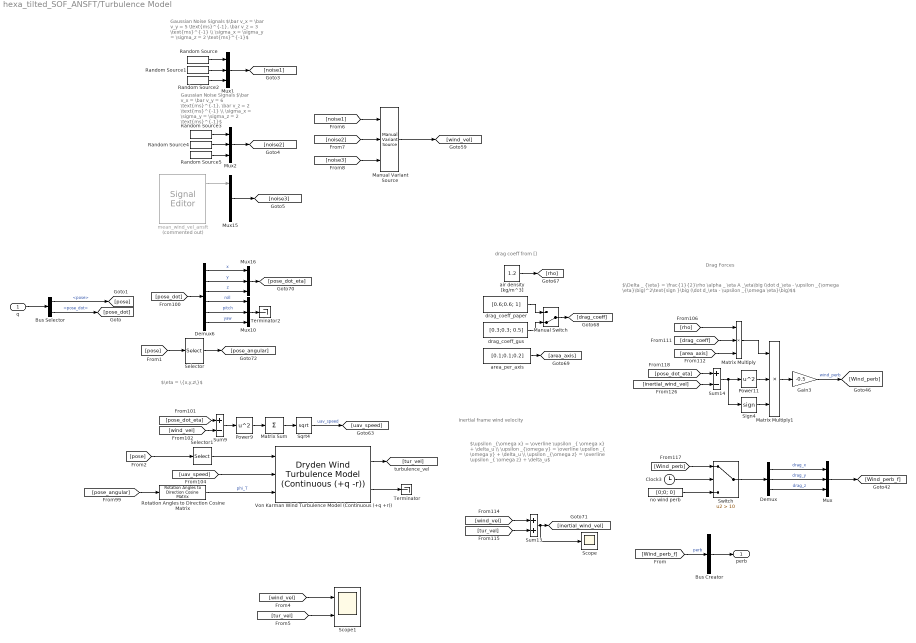
== system hexa_tilted_SOF_ANSFT/Turbulence Model ==
  note: Gaussian Noise Signals
      | $\bar v_x = \bar v_y = 6 \text{ms}^{-1}, \bar v_z = 2 \text{ms}^{-1} \\ \sigma_x = \sigma_y = \sigma_z = 2 \text{ms}^{-1}$
  note: Gaussian Noise Signals
      | $\bar v_x = \bar v_y = 5 \text{ms}^{-1}, \bar v_z = 3 \text{ms}^{-1} \\ \sigma_x = \sigma_y = \sigma_z = 2 \text{ms}^{-1}$
  note: $\Delta _ {\eta} = \frac{1}{2}\rho \alpha _ \eta A _\eta\big (\dot d_\eta - \upsilon _{\omega \eta}\big)^2\text{sign }\big (\dot d_\eta - \upsilon _{\omega \eta}\big)$$
  note: drag coeff from []
  note: $\upsilon _{\omega x} = \overline \upsilon _{ \omega x} + \delta_u \\ \upsilon _{\omega y} = \overline \upsilon _{ \omega y} + \delta_u \\ \upsilon _{\omega z} = \overline \upsilon _{ \omega z} + \delta_u$
  note: $\eta = \{x,y,z\}$
  note: Drag Forces
  note: Inertial frame wind velocity
  q : Inport
  Bus Creator : BusCreator  Inputs=1
  Bus Selector : BusSelector  OutputSignals=pose,pose_dot
  Clock3 : Clock
  Demux : Demux  Outputs=3
  Demux6 : Demux  Outputs=6
  Gain3 : Gain  Gain=-0.5
  Manual Variant Source : simulink/Signal Routing/Manual Variant Source  NumChoices=3  LabelModeActiveChoice=V_1
  Manual Switch : ManualSwitch  CurrentSetting=0
  Matrix Sum : Sum  Inputs=+
  Matrix Multiply : Product  Inputs=3
  Matrix Multiply1 : Product  Inputs=3
  Mux{,1..2,10,15..16} (6 alike) : Mux  Inputs=3
  Power11 : Math  Operator=square
  Power9 : Math  Operator=square
  Random Source : dspsrcs4/Random Source  SrcType=Gaussian  NormMethod=Ziggurat  CltLength=12  MinVal=0  MaxVal=1  MeanVal=5  VarVal=2  RepMode=Not repeatable  rawSeed=1  IsInherit=off  SampMode=Discrete  SampTime=1  SampFrame=1  DataType=Double  OutComplex=Real  OutputFrames=off
  Random Source1 : dspsrcs4/Random Source  SrcType=Gaussian  NormMethod=Ziggurat  CltLength=12  MinVal=0  MaxVal=1  MeanVal=5  VarVal=2  RepMode=Not repeatable  rawSeed=1  IsInherit=off  SampMode=Discrete  SampTime=1  SampFrame=1  DataType=Double  OutComplex=Real  OutputFrames=off
  Random Source2 : dspsrcs4/Random Source  SrcType=Gaussian  NormMethod=Ziggurat  CltLength=12  MinVal=0  MaxVal=1  MeanVal=3  VarVal=2  RepMode=Not repeatable  rawSeed=1  IsInherit=off  SampMode=Discrete  SampTime=1  SampFrame=1  DataType=Double  OutComplex=Real  OutputFrames=off
  Random Source3 : dspsrcs4/Random Source  SrcType=Gaussian  NormMethod=Ziggurat  CltLength=12  MinVal=0  MaxVal=1  MeanVal=6  VarVal=2  RepMode=Not repeatable  rawSeed=1  IsInherit=off  SampMode=Discrete  SampTime=1  SampFrame=1  DataType=Double  OutComplex=Real  OutputFrames=off
  Random Source4 : dspsrcs4/Random Source  SrcType=Gaussian  NormMethod=Ziggurat  CltLength=12  MinVal=0  MaxVal=1  MeanVal=6  VarVal=2  RepMode=Not repeatable  rawSeed=1  IsInherit=off  SampMode=Discrete  SampTime=1  SampFrame=1  DataType=Double  OutComplex=Real  OutputFrames=off
  Random Source5 : dspsrcs4/Random Source  SrcType=Gaussian  NormMethod=Ziggurat  CltLength=12  MinVal=0  MaxVal=1  MeanVal=2  VarVal=2  RepMode=Not repeatable  rawSeed=1  IsInherit=off  SampMode=Discrete  SampTime=1  SampFrame=1  DataType=Double  OutComplex=Real  OutputFrames=off
  Rotation Angles to Direction Cosine Matrix : sharedtransform/Rotation Angles to Direction Cosine Matrix  rotationOrder=XYZ  aMode=aMode
  Scope : Scope
  Scope1 : Scope  NumInputPorts=2
  Selector : Selector  InputPortWidth=6  IndexOptions=Index vector (dialog)  Indices=[4:6]  OutputSizes=1
  Selector1 : Selector  InputPortWidth=6  IndexOptions=Index vector (dialog)  Indices=[3]  OutputSizes=1
  Sign4 : Signum
  Sqrt4 : Sqrt
  Sum13 : Sum
  Sum14 : Sum  Inputs=+-
  Sum9 : Sum  Inputs=+-
  Switch : Switch  Criteria=u2 > Threshold  Threshold=10  SaturateOnIntegerOverflow=off  InputSameDT=off
  Terminator : Terminator
  Terminator2 : Terminator
  Von Karman Wind Turbulence Model (Continuous (+q +r)) : aerolibwind2/Dryden Wind Turbulence Model  (Continuous (+q -r))  units=Metric (MKS)  spec=MIL-F-8785C  model=Continuous Von Karman (+q -r)  W20=15  Wdeg=0  TurbProb=10^-2 - Light  L_high=762  Wingspan=10  ts=0.1  Seed=[23341 23342 23343 23344]  T_on=on
      settings: LibrarySourceBlock=|
      | aerolibwind2/Von Karman Wind Turbulence Model
      | (Continuous (+q +r))
  air density [kg/m^3] : Constant  Value=1.2
  area_per_axis : Constant  Value=[0.1;0.1;0.2]
  drag_coeff_gus : Constant  Value=[0.3;0.3; 0.5]
  drag_coeff_paper : Constant  Value=[0.6;0.6; 1]
  mean_wind_vel_ansft : SignalEditorBlockLib/Signal Editor  Commented=on  FileName=mean_wind_vel_ansft.mat  ActiveScenario=Velocidades_medias_del_viento  ActiveSignal=wean_wind_vel_x  IsBus=off  OutputBusObjectStr=Bus: BusObject  SampleTime=0  Interpolate=off  ZeroCross=off  OutputAfterFinalValue=Setting to zero  Unit=inherit  PreserveSignalName=on  ApplySigPropsToAllScenarios=on
  no wind perb : Constant  Value=[0;0; 0]
  perb : Outport
  wires:
  Demux6/1 -> Mux16/1  "x"
  [rho] -> Matrix Multiply/1
  Demux6/3 -> Mux16/3  "z"
  Manual Switch/1 -> [drag_coeff]
  Power11/1 -> Matrix Multiply1/2
  Von Karman Wind Turbulence Model (Continuous (+q +r))/1 -> [tur_vel]
  Rotation Angles to Direction Cosine Matrix/1 -> Von Karman Wind Turbulence Model (Continuous (+q +r))/3  "phi_T"
  drag_coeff_paper/1 -> Manual Switch/1
  Matrix Sum/1 -> Sqrt4/1
  Gain3/1 -> [Wind_perb]  "wind_perb"
  Matrix Multiply/1 -> Matrix Multiply1/1
  Selector/1 -> [pose_angular]
  Sum9/1 -> Power9/1
  no wind perb/1 -> Switch/3
  Mux16/1 -> [pose_dot_eta]
  Clock3/1 -> Switch/2
  Sum14/1 -> Sign4/1, Power11/1
  [area_axis] -> Matrix Multiply/3
  Von Karman Wind Turbulence Model (Continuous (+q +r))/2 -> Terminator/1
  [uav_speed] -> Von Karman Wind Turbulence Model (Continuous (+q +r))/2
  Demux6/4 -> Mux10/1  "roll"
  [drag_coeff] -> Matrix Multiply/2
  air density [kg/m^3]/1 -> [rho]
  Mux10/1 -> Terminator2/1
  area_per_axis/1 -> [area_axis]
  [pose_angular] -> Rotation Angles to Direction Cosine Matrix/1
  drag_coeff_gus/1 -> Manual Switch/2
  Sum13/1 -> Scope/1, [inertial_wind_vel]
  Switch/1 -> Demux/1
  [pose_dot_eta] -> Sum9/1
  Demux6/5 -> Mux10/2  "pitch"
  [tur_vel] -> Sum13/2
  Selector1/1 -> Von Karman Wind Turbulence Model (Continuous (+q +r))/1
  [pose_dot_eta] -> Sum14/1
  [wind_vel] -> Sum9/2
  [Wind_perb] -> Switch/1
  [wind_vel] -> Sum13/1
  Sqrt4/1 -> [uav_speed]  "uav_speed"
  Demux6/6 -> Mux10/3  "yaw"
  Sign4/1 -> Matrix Multiply1/3
  Demux6/2 -> Mux16/2  "y"
  Power9/1 -> Matrix Sum/1
  Matrix Multiply1/1 -> Gain3/1
  [pose_dot] -> Demux6/1
  [inertial_wind_vel] -> Sum14/2
  Bus Creator/1 -> perb/1
  [Wind_perb_f] -> Bus Creator/1  "perb"
  q/1 -> Bus Selector/1
  Bus Selector/2 -> [pose_dot]  "<pose_dot>"
  Bus Selector/1 -> [pose]  "<pose>"
  [pose] -> Selector/1
  [pose] -> Selector1/1
  mean_wind_vel_ansft/1 -> Mux15/1
  Demux/1 -> Mux/1  "drag_x"
  Demux/2 -> Mux/2  "drag_y"
  Demux/3 -> Mux/3  "drag_z"
  Mux/1 -> [Wind_perb_f]
  [wind_vel] -> Scope1/1
  [tur_vel] -> Scope1/2
  Random Source/1 -> Mux1/1
  Random Source1/1 -> Mux1/2
  Random Source2/1 -> Mux1/3
  Mux1/1 -> [noise1]
  Random Source4/1 -> Mux2/2
  Random Source5/1 -> Mux2/3
  Random Source3/1 -> Mux2/1
  Mux2/1 -> [noise2]
  Mux15/1 -> [noise3]
  Manual Variant Source/1 -> [wind_vel]
  [noise2] -> Manual Variant Source/2
  [noise3] -> Manual Variant Source/3
  [noise1] -> Manual Variant Source/1
  ? -> Mux15/2
  ? -> Mux15/3

== matlab function hexa_tilted_SOF_ANSFT/Trajectory/Helicoidal Trajectory ==
  data: time input; pose_d output; pose_d_dot output; pose_d_ddot output
function [pose_d, pose_d_dot, pose_d_ddot]= fcn(time)

% pos_z = time / 12;
f = 0.15;
arg = f * (time - 5);
r = 2;

% hover for 5 s | include inclination in roll
% 5 metros al menos

roll = 0;
% yaw = pi / 2;
yaw = 0;

if (time < 5)
    pos_x = 0;
    pos_y = 0;
    % roll = 0;
    pos_z = 0.4 * time;
    % yaw = 0;
else
    pos_x = -r + r * cos (arg);
    pos_y = r * sin (arg);
    pos_z = 2;
    % roll = 0.15;
    % yaw = (time - 5) * 2 * pi / 180; 
end

% roll = 0;
% yaw = time * 0;

pose_d = [pos_x;
          pos_y;
          pos_z;
          roll;
          0;
          yaw];

% pos_z_dot = 1 / 12;

% hover for 5 s
if (time < 5)
    pos_x_dot = 0;
    pos_y_dot = 0;
    pos_z_dot = 0.4;
    % yaw_dot = 0;
else
    pos_x_dot = - f * r * sin(arg);
    pos_y_dot = f * r * cos(arg);
    pos_z_dot = 0;
    % yaw_dot = 2 * pi / 180;
end

yaw_dot = 0;

pose_d_dot = [pos_x_dot;
              pos_y_dot;
              pos_z_dot;
              0;
              0;
              yaw_dot];

pos_z_ddot = 0;
% hover for 5 s
if (time < 5)
    pos_x_ddot = 0;
    pos_y_ddot = 0;
else
    pos_x_ddot = - f * f * r * cos(arg);
    pos_y_ddot = - f * f * r * sin(arg);
end

pose_d_ddot = [pos_x_ddot;
               pos_y_ddot;
               pos_z_ddot;
               0;
               0;
               0];

== matlab function hexa_tilted_SOF_ANSFT/Controller/ansftConstants ==
  data: xi1 output; xi2 output; lambda1 output; lambda2 output; alpha output; beta output; unused input
function [xi1, xi2, lambda1, lambda2, alpha, beta] = fcn(~)

%% Constantes de la Superficie deslizante
% zeta1 parecido a una ganancia proporcional
xi1 = [3; 3; 1.5; 5; 5; 2];
%zeta2 parecido a una ganancia derivatida
xi2 = [1; 1; 1.25; 0.5; 0.5; 1];
% lambda 1 > lambda2
lambda1 = [2.5; 2.5; 1.75; 2.5; 2.5; 2];
% 1 < lambda2 < 2
lambda2 = [1.25; 1.25; 1.25; 1.33; 1.33; 1.2];

%% Constantes del control auxiliar
%minimize sigma
alpha = [1.25; 1.25; 1.25; 3.75; 3.75; 1.25];

%aumetnar control, aumentar energía del sistema
beta = [1.5; 1.5; 0.75; 0.5; 0.5; 1.2];

== matlab function hexa_tilted_SOF_ANSFT/6DoF-Dynamics/calculatePhiMatrix ==
  data: Phi output; M output; M_inv output; v input; m input
function [Phi, M, M_inv] = fcn(v, m)

% Jxx =  24778420.82/(1000*1000000); % kg m²
% Jyy = 42217933.96/(1000*1000000); % kg m²
% Jzz = 23948304.24/(1000*1000000); % kg m²
Jxx = 0.0374;
Jyy = 0.0385;
Jzz = 0.0593;
%% Phi matrix calculation
uu = v(1);
vv = v(2);
ww = v(3);
pp = v(4);
qq = v(5);
rr = v(6);


Phi = [0, -rr, qq, 0, -ww, vv;
        rr, 0, -pp , ww, 0, -uu;
        -qq, pp, 0,  -vv, uu, 0;
        0, 0, 0, 0, -rr, qq; 
        0, 0, 0, rr, 0, -pp;
        0, 0, 0, -qq, pp, 0];

Phi = transpose(Phi);

M = [m, 0, 0, 0, 0, 0;
    0, m, 0, 0, 0, 0;
    0, 0, m, 0, 0, 0;
    0, 0, 0, Jxx, 0, 0;
    0, 0, 0, 0, Jyy, 0;
    0, 0, 0, 0, 0, Jzz];

M_inv = inv(M);

%% Fg matrix calculation

== matlab function hexa_tilted_SOF_ANSFT/Trajectory/Lemniscate Trajectory ==
  data: time input; pose_d output; pose_d_dot output; pose_d_ddot output
function [pose_d, pose_d_dot, pose_d_ddot]= fcn(time)

%% Positions

arg = time / 4;
rx = 2;
ry = 2;

pos_x = rx * sin(arg);
pos_y = ry * sin(arg) * cos(arg);
pos_z = 0;

yaw = time * 0;

pose_d = [pos_x;
          pos_y;
          pos_z;
          0;
          0;
          yaw];

%% Velocities

pos_x_dot = rx * 0.25 * cos(arg);
pos_y_dot = ry * 0.25 * cos(2 * arg);
pos_z_dot = 0;
yaw_dot = 0;

pose_d_dot = [pos_x_dot;
              pos_y_dot;
              pos_z_dot;
              0;
              0;
              yaw_dot];

%% Accelerations

pos_x_ddot = - rx * 0.25 * 0.25 * sin(arg);
pos_y_ddot = - ry * 0.25 * 0.25 * 2 * sin(arg);
pos_z_ddot = 0;
yaw_ddot = 0;

pose_d_ddot = [pos_x_ddot;
               pos_y_ddot;
               pos_z_ddot;
               0;
               0;
               yaw_ddot];

== matlab function hexa_tilted_SOF_ANSFT/6DoF-Dynamics/calculateRotationMatrix ==
  data: pose input; Rib output
function Rib  = fcn(pose)

roll = pose(4);
pitch = pose(5);
yaw = pose(6);

R1 = [cos(yaw)*cos(pitch), -cos(roll)*sin(yaw) + cos(yaw)*sin(roll)*sin(pitch), sin(roll)*sin(yaw) + cos(roll)*cos(yaw)*sin(pitch);
       cos(pitch)*sin(yaw), cos(roll)*cos(yaw) + sin(yaw)*sin(pitch)*sin(roll), -cos(yaw)*sin(roll) + sin(yaw)*sin(pitch)*cos(roll);
       -sin(pitch), cos(pitch)*sin(roll), cos(pitch)*cos(roll)];

R2 = [1, sin(roll)*tan(pitch), cos(roll)*tan(pitch);
      0, cos(roll), -sin(roll);
      0, sin(roll)/cos(pitch), cos(roll)/cos(pitch)];

Rzeros = zeros(3);

Rib = [R1, Rzeros;
       Rzeros, R2];

== matlab function hexa_tilted_SOF_ANSFT/Controller/calculatePWM ==
  data: omega2 input; pwm output
function pwm = fcn(omega2)

pwm = -1.3121e-09 .* omega2 .* omega2 + 0.00208 .* omega2 + 1107.922;

== matlab function hexa_tilted_SOF_ANSFT/6DoF-Dynamics/calculateGravityVector ==
  data: m input; pose input; Fg output
function Fg  = fcn(m, pose)

g = 9.81;

roll = pose(4);
pitch = pose(5);

Fg = [m*g*sin(pitch);
      -m*g*cos(pitch)*sin(roll);
      -m*g*cos(pitch)*cos(roll);
      0;
      0;
      0];

== matlab function hexa_tilted_SOF_ANSFT/SecondOrderFilter/SOF_gains ==
  data: omega_n output
function omega_n = fcn

omega_n = [30; 30; 50; 50; 50; 50];

== matlab function hexa_tilted_SOF_ANSFT/Controller/calculatePhiMatrix ==
  data: Phi output; v input
function Phi  = fcn(v)

% Jxx =  24778420.82/(1000*1000000); % kg m²
% Jyy = 42217933.96/(1000*1000000); % kg m²
% Jzz = 23948304.24/(1000*1000000); % kg m²
Jxx = 0.0374;
Jyy = 0.0385;
Jzz = 0.0593;
%% Phi matrix calculation
uu = v(1);
vv = v(2);
ww = v(3);
pp = v(4);
qq = v(5);
rr = v(6);


Phi = [0, -rr, qq, 0, -ww, vv;
        rr, 0, -pp , ww, 0, -uu;
        -qq, pp, 0,  -vv, uu, 0;
        0, 0, 0, 0, -rr, qq; 
        0, 0, 0, rr, 0, -pp;
        0, 0, 0, -qq, pp, 0];

Phi = transpose(Phi);

== matlab function hexa_tilted_SOF_ANSFT/Controller/calculateRotationMatrix ==
  data: pose input; Rbi output
function Rbi  = fcn(pose)

roll = pose(4);
pitch = pose(5);
yaw = pose(6);

R1 = [cos(yaw)*cos(pitch), -cos(roll)*sin(yaw) + cos(yaw)*sin(roll)*sin(pitch), sin(roll)*sin(yaw) + cos(roll)*cos(yaw)*sin(pitch);
       cos(pitch)*sin(yaw), cos(roll)*cos(yaw) + sin(yaw)*sin(pitch)*sin(roll), -cos(yaw)*sin(roll) + sin(yaw)*sin(pitch)*cos(roll);
       -sin(pitch), cos(pitch)*sin(roll), cos(pitch)*cos(roll)];

R2 = [1, sin(roll)*tan(pitch), cos(roll)*tan(pitch);
      0, cos(roll), -sin(roll);
      0, sin(roll)/cos(pitch), cos(roll)/cos(pitch)];

Rzeros = zeros(3);

Rbi = [transpose(R1), Rzeros;
       Rzeros, inv(R2)];
